simulink model "Singularities_G18"  (R2016a)
settings: Solver=VariableStepAuto  SolverMode=SingleTasking  StartTime=0.0  StopTime=inf  RelTol=1e-3
libraries: vrlib x7
settings Model: Creator=Ricardo Henriques  LastModifiedBy=Catarina
settings DebuggingCC: SFUnexpectedBacktrackingDiag=error  SFNoUnconditionalDefaultTransitionDiag=error
settings GRTTargetCC: TargetLangStandard=C99 (ISO)  GeneratePreprocessorConditionals=Use local settings
settings ConfigComp: CovMetricSettings=dwe  CovHtmlReporting=off  CovSaveCumulativeToWorkspaceVar=off  CovSaveSingleToWorkspaceVar=off  CovExternalEMLEnable=on

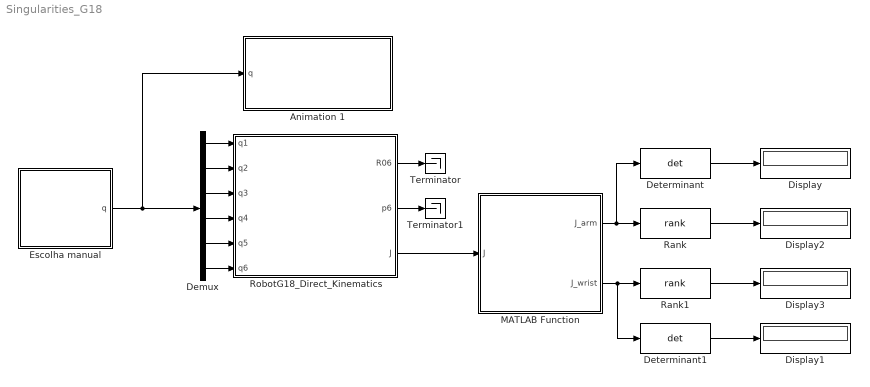
== system Singularities_G18 ==
  Animation 1 : Subsystem
  Demux : Demux  Outputs=6
  Determinant : MATLABFcn  MATLABFcn=det
  Determinant1 : MATLABFcn  MATLABFcn=det
  Display{,1..3} (4 alike) : Display
  "Escolha manual " : Subsystem  mask{q1=-104.400, q2=18.0, q3=10.800, q4=-147.600, q5=-3.600, q6=-79.200}
  MATLAB Function : MATLAB Function  TreatAsAtomicUnit=on
  Rank : MATLABFcn  MATLABFcn=rank
  Rank1 : MATLABFcn  MATLABFcn=rank
  RobotG18_Direct_Kinematics : MATLAB Function  TreatAsAtomicUnit=on
  Terminator : Terminator
  Terminator1 : Terminator
  wires:
  RobotG18_Direct_Kinematics/1(R06) -> Terminator/1
  RobotG18_Direct_Kinematics/3(J) -> MATLAB Function/1(J)
  Demux/1 -> RobotG18_Direct_Kinematics/1(q1)
  Demux/2 -> RobotG18_Direct_Kinematics/2(q2)
  Demux/3 -> RobotG18_Direct_Kinematics/3(q3)
  Demux/4 -> RobotG18_Direct_Kinematics/4(q4)
  Demux/5 -> RobotG18_Direct_Kinematics/5(q5)
  Demux/6 -> RobotG18_Direct_Kinematics/6(q6)
  MATLAB Function/1(J_arm) -> Determinant/1, Rank/1
  MATLAB Function/2(J_wrist) -> Determinant1/1, Rank1/1
  "Escolha manual "/1("q ") -> Animation 1/1("q "), Demux/1
  RobotG18_Direct_Kinematics/2(p6) -> Terminator1/1
  Rank/1 -> Display2/1
  Rank1/1 -> Display3/1
  Determinant/1 -> Display/1
  Determinant1/1 -> Display1/1

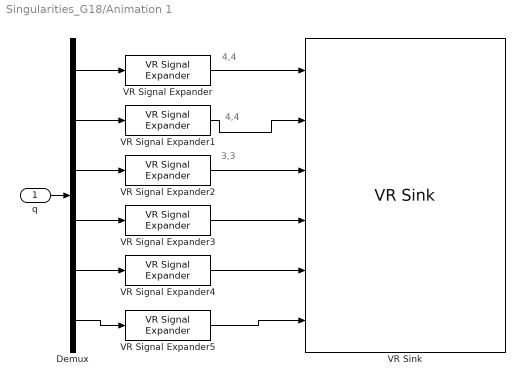
== system Singularities_G18/Animation 1 ==
  note: 4,4
  note: 3,3
  note: 4,4
  "q " : Inport
  Demux : Demux  Outputs=6
  VR Signal Expander{,1..5} (6 alike) : vrlib/VR Signal Expander  outwidth=4  outidx=4
  VR Sink : vrlib/VR Sink  InstantiateOnLoad=on  SampleTime=0.1  ViewEnable=on  RemoteChange=off  RemoteView=off  FieldsWritten=Jt1_DH_dv.rotation.4.1.1.double#Jt2_DH_dv.rotation.4.1.1.double#Jt3_DH_dv.rotation.4.1.1.double#Jt4_DH_dv.rotation.4.1.1.double#Jt5_DH_dv.rotation.4.1.1.double#Jt6_DH_dv.rotation.4.1.1.double  WorldFileName=RobotG18_Opt_NoAxes.wrl  WorldDescription=D-H Reference Frames for Virtual Reality Robot  AutoView=off  VideoDimensions=[]  AllowVariableSize=off
  wires:
  "q "/1 -> Demux/1
  Demux/1 -> VR Signal Expander/1
  Demux/2 -> VR Signal Expander1/1
  Demux/3 -> VR Signal Expander2/1
  Demux/4 -> VR Signal Expander3/1
  Demux/5 -> VR Signal Expander4/1
  Demux/6 -> VR Signal Expander5/1
  VR Signal Expander/1 -> VR Sink/1
  VR Signal Expander1/1 -> VR Sink/2
  VR Signal Expander5/1 -> VR Sink/6
  VR Signal Expander2/1 -> VR Sink/3
  VR Signal Expander3/1 -> VR Sink/4
  VR Signal Expander4/1 -> VR Sink/5

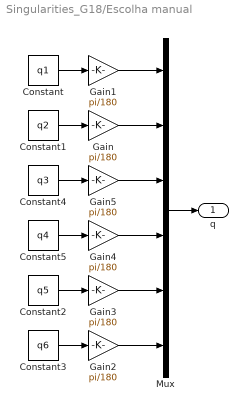
== system Singularities_G18/Escolha manual  ==
  Constant : Constant  Value=q1
  Constant1 : Constant  Value=q2
  Constant2 : Constant  Value=q5
  Constant3 : Constant  Value=q6
  Constant4 : Constant  Value=q3
  Constant5 : Constant  Value=q4
  Gain{,1..5} (6 alike) : Gain  Gain=pi/180
  Mux : Mux  Inputs=6
  "q " : Outport
  wires:
  Constant/1 -> Gain1/1
  Constant1/1 -> Gain/1
  Mux/1 -> "q "/1
  Gain1/1 -> Mux/1
  Gain/1 -> Mux/2
  Constant2/1 -> Gain3/1
  Constant3/1 -> Gain2/1
  Constant4/1 -> Gain5/1
  Constant5/1 -> Gain4/1
  Gain5/1 -> Mux/3
  Gain4/1 -> Mux/4
  Gain3/1 -> Mux/5
  Gain2/1 -> Mux/6

== matlab function Singularities_G18/MATLAB Function ==
  data: J input; J_arm output; J_wrist output
function [J_arm, J_wrist] = ArmAndWrist(J)
J_arm = J(1:3,1:3);
J_wrist = J(4:6,4:6);
J_arm = double(J_arm);
J_wrist = double(J_wrist);
end

== matlab function Singularities_G18/RobotG18_Direct_Kinematics ==
  data: q1 input; R06 output; q2 input; q3 input; q4 input; q5 input; q6 input; p6 output; J output
function [R06,p6,J] = RobotG18_Direct_Kinematics(q1,q2,q3,q4,q5,q6)
%#codegen

%    This function was generated by the Symbolic Math Toolbox version 7.0.
%    15-Apr-2021 18:49:51

t2 = q2+q3+q4;
t3 = cos(q1);
t4 = sin(q6);
t5 = sin(q1);
t6 = sin(q5);
t7 = t5.*t6;
t8 = cos(t2);
t9 = cos(q5);
t10 = t7-t3.*t8.*t9;
t11 = sin(t2);
t12 = cos(q6);
t13 = t3.*t6;
t14 = t5.*t8.*t9;
t15 = t13+t14;
t16 = q2+q3;
t17 = cos(q2);
t18 = sin(q2);
t19 = sin(q3);
t20 = cos(t16);
t21 = sin(q4);
t22 = sin(t16);
t23 = cos(q4);
t24 = cos(q3);
t25 = t5.*t17.*(1.7e1./4.0e1);
t26 = t5.*t6.*t8.*(4.1e1./5.0e2);
t27 = t5.*t17.*t24.*(4.9e1./1.25e2);
t28 = t22.*(4.9e1./1.25e2);
t29 = t18.*(1.7e1./4.0e1);
t30 = t20.*t21.*(4.1e1./5.0e2);
t31 = t22.*t23.*(4.1e1./5.0e2);
t32 = t30+t31;
t33 = t6.*t32;
t34 = t20.*t23.*(1.9e1./2.0e2);
t35 = t8.*(1.9e1./2.0e2);
t36 = t6.*t11.*(4.1e1./5.0e2);
t37 = t5.*(1.09e2./1.0e3);
t38 = t3.*t17.*(1.7e1./4.0e1);
t39 = t5.*t9.*(4.1e1./5.0e2);
t40 = t3.*t6.*t8.*(4.1e1./5.0e2);
t41 = t3.*t17.*t24.*(4.9e1./1.25e2);
t42 = t37+t38+t39+t40+t41-t3.*t18.*t19.*(4.9e1./1.25e2)-t3.*t20.*t21.*(1.9e1./2.0e2)-t3.*t22.*t23.*(1.9e1./2.0e2);
t43 = t28+t29+t33+t34-t21.*t22.*(1.9e1./2.0e2);
t44 = t28+t35+t36;
t45 = t35+t36;
t46 = q2+q3+q4+q5;
t47 = sin(t46);
t48 = t47.*(4.1e1./1.0e3);
t49 = t20.*(4.9e1./1.25e2);
t50 = q2+q3+q4-q5;
t51 = sin(t50);
t52 = t5.*t9;
t53 = t3.*t6.*t8;
t54 = t52+t53;
t55 = t5.*t6.*t8;
t56 = t55-t3.*t9;
t57 = t6.*t11;
R06 = reshape([-t10.*t12-t3.*t4.*t11,t12.*t15-t4.*t5.*t11,t4.*t8+t9.*t11.*t12,t4.*t10-t3.*t11.*t12,-t4.*t15-t5.*t11.*t12,t8.*t12-t4.*t9.*t11,t54,t56,t57],[3,3]);
if nargout > 1
    p6 = [t42;t3.*(-1.09e2./1.0e3)+t25+t26+t27-t3.*t9.*(4.1e1./5.0e2)-t5.*t18.*t19.*(4.9e1./1.25e2)-t5.*t20.*t21.*(1.9e1./2.0e2)-t5.*t22.*t23.*(1.9e1./2.0e2);t28+t29+t33+t34-t21.*t22.*(1.9e1./2.0e2)+8.9e1./1.0e3];
end
if nargout > 2
    J = reshape([t3.*(1.09e2./1.0e3)-t25-t26-t27+t3.*t9.*(4.1e1./5.0e2)+t5.*t18.*t19.*(4.9e1./1.25e2)+t5.*t20.*t21.*(1.9e1./2.0e2)+t5.*t22.*t23.*(1.9e1./2.0e2),t42,0.0,0.0,0.0,1.0,-t3.*t43,-t5.*t43,t11.*(-1.9e1./2.0e2)+t17.*(1.7e1./4.0e1)+t48+t49-t51.*(4.1e1./1.0e3),t5,-t3,0.0,-t3.*t44,-t5.*t44,t11.*(-1.9e1./2.0e2)+t48+t49-t51.*(4.1e1./1.0e3),t5,-t3,0.0,-t3.*t45,-t5.*t45,t11.*(-1.9e1./2.0e2)+t48-t51.*(4.1e1./1.0e3),t5,-t3,0.0,t5.*t6.*(-4.1e1./5.0e2)-t3.*t9.*t17.*t19.*t21.*(4.1e1./5.0e2)-t3.*t9.*t18.*t19.*t23.*(4.1e1./5.0e2)-t3.*t9.*t18.*t21.*t24.*(4.1e1./5.0e2)+t3.*t9.*t17.*t23.*t24.*(4.1e1./5.0e2),t3.*t6.*(4.1e1./5.0e2)-t5.*t9.*t17.*t19.*t21.*(4.1e1./5.0e2)-t5.*t9.*t18.*t19.*t23.*(4.1e1./5.0e2)-t5.*t9.*t18.*t21.*t24.*(4.1e1./5.0e2)+t5.*t9.*t17.*t23.*t24.*(4.1e1./5.0e2),t48+t51.*(4.1e1./1.0e3),-t3.*t11,-t5.*t11,t8,0.0,0.0,0.0,t54,t56,t57],[6,6]);
end
